simulink model "gbp_ut"  (Simulink 8.1)
settings: Solver=FixedStepDiscrete  StartTime=0.0  StopTime=Inf  FixedStep=0.005  RelTol=1e-3
libraries: siltestlib x2, gbp x1
settings Model: Creator=xsellart  LastModifiedBy=AT015555
settings DataIOCC: SignalLoggingSaveFormat=Dataset
settings OptimizationCC: ExpressionDepthLimit=128
settings DebuggingCC: FcnCallInpInsideContextMsg=EnableAllAsError
settings GRTTargetCC: CombineOutputUpdateFcns=on  GRTInterface=off

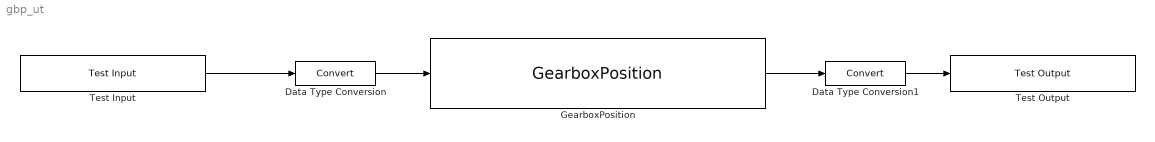
== system gbp_ut ==
  Data Type Conversion : DataTypeConversion
  Data Type Conversion1 : DataTypeConversion
  GearboxPosition : gbp/GearboxPosition
  Test Input : siltestlib/Test Input  varname=VDINR_NowGearPosn_enum  sampletime=0.005
  Test Output : siltestlib/Test Output  varname=VIFO_DriveGearPosn_flg  sampletime=-1
  wires:
  Data Type Conversion1/1 -> Test Output/1
  Test Input/1 -> Data Type Conversion/1
  Data Type Conversion/1 -> GearboxPosition/1
  GearboxPosition/1 -> Data Type Conversion1/1
